simulink model "practice"  (R2019b)
settings: Solver=VariableStepAuto  StartTime=0.0  StopTime=10.0  RelTol=1e-3
libraries: commfilt2 x3, commsink2 x2, commutil2 x2, dspindex x2, commrandsrc3 x2
settings Model: Creator=DELL  LastModifiedBy=DELL

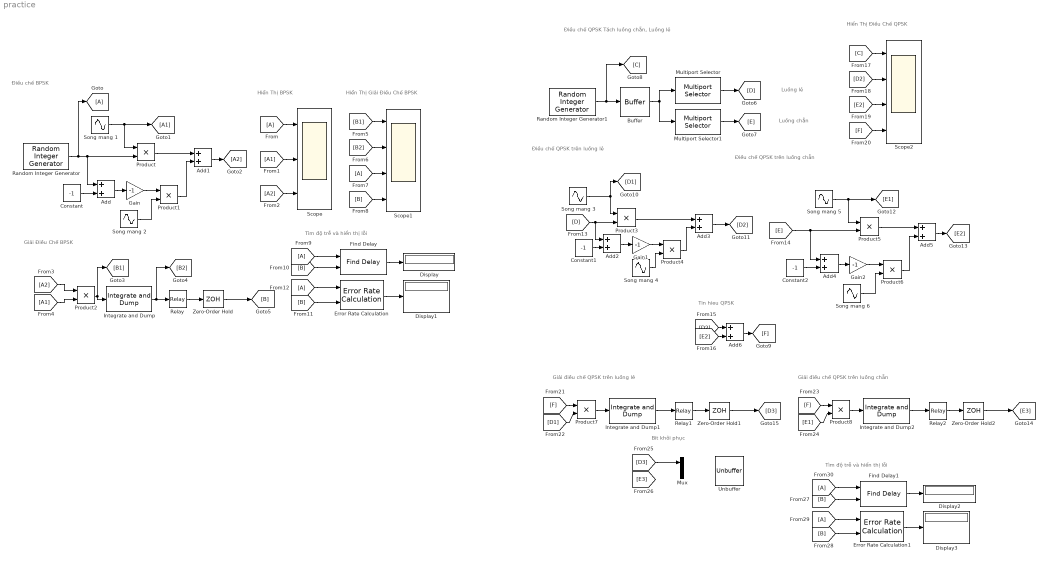
== system practice ==
  note: Luồng lẻ
  note: Điều chế BPSK
  note: Hiển Thị BPSK
  note: Hiển Thị Giải Điều Chế BPSK
  note: Giải Điều Chế BPSK
  note: Tìm độ trễ và hiển thị lỗi
  note: Điều chế QPSK
      | Tách luồng chẵn, Luồng lẻ
  note: Luồng chẵn
  note: Điều chế QPSK trên luồng lẻ
  note: Điều chế QPSK trên luồng chẵn
  note: Hiển Thị Điều Chế QPSK
  note: Tin hieu QPSK
  note: Giải điều chế QPSK trên luồng lẻ
  note: Giải điều chế QPSK trên luồng chẵn
  note: Bit khôi phục
  note: Tìm độ trễ và hiển thị lỗi
  Add{,1..6} (7 alike) : Sum
  Buffer : Buffer  N=2  OutputFrames=off
  Constant : Constant  Value=-1
  Constant1 : Constant  Value=-1
  Constant2 : Constant  Value=-1
  Display{,1..3} (4 alike) : Display
  Error Rate Calculation : commsink2/Error Rate Calculation  N=1  st_delay=0  cp_mode=Entire frame  subframe=[]  PMode=Port  WsName=ErrorVec  RsMode2=off  stop=off  numErr=100  maxBits=1e6
      settings: SourceProductName=Communications Toolbox
  Error Rate Calculation1 : commsink2/Error Rate Calculation  N=1  st_delay=0  cp_mode=Entire frame  subframe=[]  PMode=Port  WsName=ErrorVec  RsMode2=off  stop=off  numErr=100  maxBits=1e6
      settings: SourceProductName=Communications Toolbox
  Find Delay : commutil2/Find Delay  corrLength=200  chgSigOP=off  stopUpdate=off  numConstDelay=3
      settings: SourceProductName=Communications Toolbox  SourceProductBaseCode=CM
  Find Delay1 : commutil2/Find Delay  corrLength=200  chgSigOP=off  stopUpdate=off  numConstDelay=3
      settings: SourceProductName=Communications Toolbox  SourceProductBaseCode=CM
  Gain : Gain  Gain=-1
  Gain1 : Gain  Gain=-1
  Gain2 : Gain  Gain=-1
  Integrate and Dump : commfilt2/Integrate and Dump  obssamples=50  offsetsamples=0  nodump=off  roundingMode=Floor  overflowMode=off  outputDataTypeStr=Inherit: Same as accumulator  outputLastDataTypeStr=Inherit: Same as accumulator
      settings: SourceProductName=Communications Toolbox
  Integrate and Dump1 : commfilt2/Integrate and Dump  obssamples=100  offsetsamples=0  nodump=off  roundingMode=Floor  overflowMode=off  outputDataTypeStr=Inherit: Same as accumulator  outputLastDataTypeStr=Inherit: Same as accumulator
      settings: SourceProductName=Communications Toolbox
  Integrate and Dump2 : commfilt2/Integrate and Dump  obssamples=100  offsetsamples=0  nodump=off  roundingMode=Floor  overflowMode=off  outputDataTypeStr=Inherit: Same as accumulator  outputLastDataTypeStr=Inherit: Same as accumulator
      settings: SourceProductName=Communications Toolbox
  Multiport Selector : dspindex/Multiport Selector  rowsOrCols=Rows  idxCellArray={ 1}  idxErrMode=Clip Index
  Multiport Selector1 : dspindex/Multiport Selector  rowsOrCols=Rows  idxCellArray={ 2 }  idxErrMode=Clip Index
  Mux : Mux  Inputs=2
  Product{,1..8} (9 alike) : Product
  Random Integer Generator : commrandsrc3/Random Integer Generator  SetSize=2  SeedSource=Auto  Seed=0  SampleTime=1/2000  SamplesPerFrame=1  OutputDataType=double  SimulateUsing=Interpreted execution
      settings: SourceProductName=Communications Toolbox
  Random Integer Generator1 : commrandsrc3/Random Integer Generator  SetSize=2  SeedSource=Auto  Seed=0  SampleTime=1/2000  SamplesPerFrame=1  OutputDataType=double  SimulateUsing=Interpreted execution
      settings: SourceProductName=Communications Toolbox
  Relay : Relay  OnSwitchValue=0  OffSwitchValue=0
  Relay1 : Relay  OnSwitchValue=0  OffSwitchValue=0
  Relay2 : Relay  OnSwitchValue=0  OffSwitchValue=0
  Scope : Scope  NumInputPorts=3
  Scope1 : Scope  NumInputPorts=4
  Scope2 : Scope  NumInputPorts=4
  Song mang 1 : Sin  Frequency=2*pi*10000  SampleTime=1/100000
  Song mang 2 : Sin  Frequency=2*pi*10000  Phase=pi  SampleTime=1/100000
  Song mang 3 : Sin  Frequency=2*pi*10000  SampleTime=1/100000
  Song mang 4 : Sin  Frequency=2*pi*10000  Phase=pi  SampleTime=1/100000
  Song mang 5 : Sin  Frequency=2*pi*10000  Phase=pi/2  SampleTime=1/100000
  Song mang 6 : Sin  Frequency=2*pi*10000  Phase=-pi/2  SampleTime=1/100000
  Unbuffer : Unbuffer
  Zero-Order Hold : ZeroOrderHold  SampleTime=1/2000
  Zero-Order Hold1 : ZeroOrderHold  SampleTime=1/1000
  Zero-Order Hold2 : ZeroOrderHold  SampleTime=1/1000
  wires:
  Random Integer Generator/1 -> [A], Add/1, Product/2
  Song mang 1/1 -> [A1], Product/1
  Constant/1 -> Add/2
  Add/1 -> Gain/1
  Gain/1 -> Product1/1
  Song mang 2/1 -> Product1/2
  Product/1 -> Add1/1
  Product1/1 -> Add1/2
  Add1/1 -> [A2]
  [A] -> Scope/1
  [A1] -> Scope/2
  [A2] -> Scope/3
  Relay/1 -> Zero-Order Hold/1
  Integrate and Dump/1 -> [B2], Relay/1
  Zero-Order Hold/1 -> [B]
  [A] -> Scope1/3
  [B2] -> Scope1/2
  [B1] -> Scope1/1
  [B] -> Scope1/4
  [B] -> Find Delay/2
  [A] -> Find Delay/1
  [B] -> Error Rate Calculation/2
  [A] -> Error Rate Calculation/1
  Find Delay/1 -> Display/1
  Error Rate Calculation/1 -> Display1/1
  Product2/1 -> Integrate and Dump/1, [B1]
  [A2] -> Product2/1
  [A1] -> Product2/2
  Random Integer Generator1/1 -> [C], Buffer/1
  Buffer/1 -> Multiport Selector1/1, Multiport Selector/1
  Multiport Selector/1 -> [D]
  Multiport Selector1/1 -> [E]
  Add3/1 -> [D2]
  Product4/1 -> Add3/2
  Product3/1 -> Add3/1
  Song mang 4/1 -> Product4/2
  Gain1/1 -> Product4/1
  Add2/1 -> Gain1/1
  Constant1/1 -> Add2/2
  Song mang 3/1 -> Product3/1, [D1]
  [D] -> Add2/1, Product3/2
  [E] -> Add4/1, Product5/2
  Song mang 5/1 -> [E1], Product5/1
  Constant2/1 -> Add4/2
  Add4/1 -> Gain2/1
  Gain2/1 -> Product6/1
  Song mang 6/1 -> Product6/2
  Product5/1 -> Add5/1
  Product6/1 -> Add5/2
  Add5/1 -> [E2]
  [D2] -> Add6/1
  [E2] -> Add6/2
  Add6/1 -> [F]
  [F] -> Scope2/4
  [C] -> Scope2/1
  [D2] -> Scope2/2
  [E2] -> Scope2/3
  [F] -> Product7/1
  [D1] -> Product7/2
  Product7/1 -> Integrate and Dump1/1
  Zero-Order Hold1/1 -> [D3]
  Relay1/1 -> Zero-Order Hold1/1
  Integrate and Dump1/1 -> Relay1/1
  Integrate and Dump2/1 -> Relay2/1
  Relay2/1 -> Zero-Order Hold2/1
  Zero-Order Hold2/1 -> [E3]
  Product8/1 -> Integrate and Dump2/1
  [E1] -> Product8/2
  [F] -> Product8/1
  Error Rate Calculation1/1 -> Display3/1
  Find Delay1/1 -> Display2/1
  [A] -> Error Rate Calculation1/1
  [B] -> Error Rate Calculation1/2
  [A] -> Find Delay1/1
  [B] -> Find Delay1/2
  [D3] -> Mux/1
